simulink model "harmonics"  (Simulink 7.0)
settings: Solver=ode23  StartTime=0.0  StopTime=0.08  RelTol=1e-3
undefined symbols (not defined in the file): D1, Delta
libraries: powerlib x26, powerlib_extras x10
settings Model: Creator=dell  LastModifiedBy=prashik nagdive

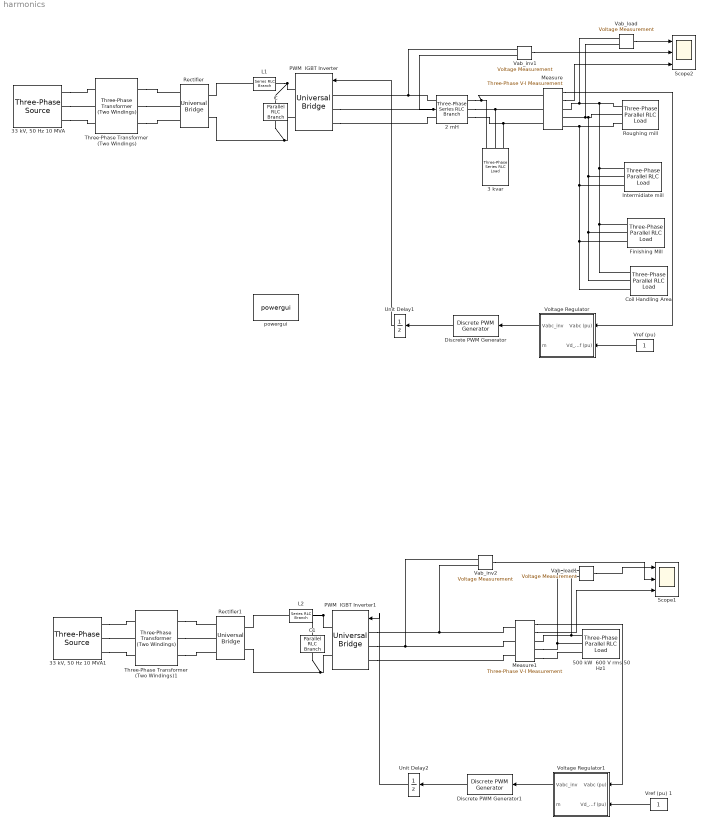
== system harmonics ==
  "2 mH " : powerlib/Elements/Three-Phase Series RLC Branch  DialogController=POWERSYS.PowerSysDialog  PhysicalDomain=powersysdomain  SubClassName=unknown  LeftPortType=p1  RightPortType=p1  LConnTagsString=A|B|C  RConnTagsString=A|B|C  BranchType=L  Resistance=1.0  Inductance=1e-3  Capacitance=1.0  Measurements=None
  3 kvar : powerlib/Elements/Three-Phase Series RLC Load  Orientation=down  DialogController=POWERSYS.PowerSysDialog  PhysicalDomain=powersysdomain  SubClassName=unknown  LeftPortType=p1  RightPortType=p1  LConnTagsString=A|B|C  Configuration=Y (grounded)  NominalVoltage=600  NominalFrequency=50  ActivePower=0  InductivePower=0  CapacitivePower=60e3  Measurements=None
  "33 kV, 50 Hz 10 MVA" : powerlib/Electrical Sources/Three-Phase Source  DialogController=POWERSYS.PowerSysDialog  SystemSampleTime=-1  Voltage=33e3  PhaseAngle=0  Frequency=50  InternalConnection=Yg  SpecifyImpedance=on  Resistance=25e3^2/10e6/5  Inductance=25e3^2/10e6/377  ShortCircuitLevel=10e6  BaseVoltage=33e3  XRratio=5
  "33 kV, 50 Hz 10 MVA1" : powerlib/Electrical Sources/Three-Phase Source  DialogController=POWERSYS.PowerSysDialog  SystemSampleTime=-1  Voltage=33e3  PhaseAngle=0  Frequency=50  InternalConnection=Yg  SpecifyImpedance=on  Resistance=25e3^2/10e6/5  Inductance=25e3^2/10e6/377  ShortCircuitLevel=10e6  BaseVoltage=33e3  XRratio=5
  500 kW  600 V rms 50 Hz1 : powerlib/Elements/Three-Phase Parallel RLC Load  DialogController=POWERSYS.PowerSysDialog  PhysicalDomain=powersysdomain  SubClassName=unknown  LeftPortType=p1  RightPortType=p1  LConnTagsString=A|B|C  Configuration=Y (grounded)  NominalVoltage=600  NominalFrequency=50  ActivePower=500e3  InductivePower=0  CapacitivePower=0  Measurements=Branch voltages and currents
  C : powerlib/Elements/Parallel RLC Branch  Orientation=down  DialogController=POWERSYS.PowerSysDialog  PhysicalDomain=powersysdomain  SubClassName=unknown  LeftPortType=p1  RightPortType=p1  LConnTagsString=a  RConnTagsString=__new0  BranchType=C  Resistance=1.0  Inductance=1.0  SetiL0=off  InitialCurrent=0  Capacitance=5000e-06  Setx0=off  InitialVoltage=0  Measurements=None
  C1 : powerlib/Elements/Parallel RLC Branch  Orientation=down  DialogController=POWERSYS.PowerSysDialog  PhysicalDomain=powersysdomain  SubClassName=unknown  LeftPortType=p1  RightPortType=p1  LConnTagsString=a  RConnTagsString=__new0  BranchType=C  Resistance=1.0  Inductance=1.0  SetiL0=off  InitialCurrent=0  Capacitance=5000e-06  Setx0=off  InitialVoltage=0  Measurements=None
  "Coil Handling Area " : powerlib/Elements/Three-Phase Parallel RLC Load  DialogController=POWERSYS.PowerSysDialog  PhysicalDomain=powersysdomain  SubClassName=unknown  LeftPortType=p1  RightPortType=p1  LConnTagsString=A|B|C  Configuration=Y (grounded)  NominalVoltage=600  NominalFrequency=50  ActivePower=500e3  InductivePower=0  CapacitivePower=0  Measurements=Branch voltages and currents
  Discrete PWM Generator : powerlib_extras/Discrete  Control Blocks/Discrete PWM Generator  Orientation=left  DialogController=POWERSYS.PowerSysDialog  SystemSampleTime=-1  GeneratorMode="3-arm  bridge (6 pulses)"  Fc=2000  Ts=2e-006  Internal=off  mIndex=0.4  Freq=60  Phase=0
  Discrete PWM Generator1 : powerlib_extras/Discrete  Control Blocks/Discrete PWM Generator  Orientation=left  DialogController=POWERSYS.PowerSysDialog  SystemSampleTime=-1  GeneratorMode="3-arm  bridge (6 pulses)"  Fc=2000  Ts=2e-006  Internal=off  mIndex=0.4  Freq=60  Phase=0
  "Finishing Mill " : powerlib/Elements/Three-Phase Parallel RLC Load  DialogController=POWERSYS.PowerSysDialog  PhysicalDomain=powersysdomain  SubClassName=unknown  LeftPortType=p1  RightPortType=p1  LConnTagsString=A|B|C  Configuration=Y (grounded)  NominalVoltage=600  NominalFrequency=50  ActivePower=500e3  InductivePower=0  CapacitivePower=0  Measurements=Branch voltages and currents
  Intermidiate mill : powerlib/Elements/Three-Phase Parallel RLC Load  DialogController=POWERSYS.PowerSysDialog  PhysicalDomain=powersysdomain  SubClassName=unknown  LeftPortType=p1  RightPortType=p1  LConnTagsString=A|B|C  Configuration=Y (grounded)  NominalVoltage=600  NominalFrequency=50  ActivePower=500e3  InductivePower=0  CapacitivePower=0  Measurements=Branch voltages and currents
  L1 : powerlib/Elements/Series RLC Branch  DialogController=POWERSYS.PowerSysDialog  PhysicalDomain=powersysdomain  SubClassName=unknown  LeftPortType=p1  RightPortType=p1  LConnTagsString=__new0  RConnTagsString=__new0  BranchType=L  Resistance=1.0  Inductance=200e-6  SetiL0=off  InitialCurrent=0  Capacitance=1.0  Setx0=off  InitialVoltage=0  Measurements=None
  L2 : powerlib/Elements/Series RLC Branch  DialogController=POWERSYS.PowerSysDialog  PhysicalDomain=powersysdomain  SubClassName=unknown  LeftPortType=p1  RightPortType=p1  LConnTagsString=__new0  RConnTagsString=__new0  BranchType=L  Resistance=1.0  Inductance=200e-6  SetiL0=off  InitialCurrent=0  Capacitance=1.0  Setx0=off  InitialVoltage=0  Measurements=None
  Measure : powerlib/Measurements/Three-Phase V-I Measurement  DialogController=POWERSYS.PowerSysDialog  SystemSampleTime=-1  VoltageMeasurement=phase-to-ground  SetLabelV=off  LabelV=V1  Vpu=on  CurrentMeasurement=yes  SetLabelI=off  LabelI=I1  Ipu=on  Pbase=500e3  Vbase=600  OutputType=Magnitude  PhasorSimulation=off  PSBequivalent=0
  Measure1 : powerlib/Measurements/Three-Phase V-I Measurement  DialogController=POWERSYS.PowerSysDialog  SystemSampleTime=-1  VoltageMeasurement=phase-to-ground  SetLabelV=off  LabelV=V1  Vpu=on  CurrentMeasurement=yes  SetLabelI=off  LabelI=I1  Ipu=on  Pbase=500e3  Vbase=600  OutputType=Magnitude  PhasorSimulation=off  PSBequivalent=0
  PWM  IGBT Inverter : powerlib/Power Electronics/Universal Bridge  Orientation=left  DialogController=POWERSYS.PowerSysDialog  SystemSampleTime=-1  Arms=3  SnubberResistance=5000  SnubberCapacitance=inf  Device=IGBT / Diodes  Ron=1e-3  Lon=0  ForwardVoltages="[  0.0  0.0  ]"  ForwardVoltage=.8  GTOparameters=[ 1e-6 ,1e-6 ]  IGBTparameters=[ 1e-6 , 2e-6 ]  Measurements=Device currents  converterType=Rectifier
  PWM  IGBT Inverter1 : powerlib/Power Electronics/Universal Bridge  Orientation=left  DialogController=POWERSYS.PowerSysDialog  SystemSampleTime=-1  Arms=3  SnubberResistance=5000  SnubberCapacitance=inf  Device=IGBT / Diodes  Ron=1e-3  Lon=0  ForwardVoltages="[  0.0  0.0  ]"  ForwardVoltage=.8  GTOparameters=[ 1e-6 ,1e-6 ]  IGBTparameters=[ 1e-6 , 2e-6 ]  Measurements=Device currents  converterType=Rectifier
  Rectifier : powerlib/Power Electronics/Universal Bridge  DialogController=POWERSYS.PowerSysDialog  SystemSampleTime=-1  Arms=3  SnubberResistance=100  SnubberCapacitance=0.1e-6  Device=Diodes  Ron=1e-3  Lon=0  ForwardVoltages="[  0.8  0.8  ]"  ForwardVoltage=.8  GTOparameters=[ 10e-6 , 20e-6 ]  IGBTparameters=[ 1e-6 , 2e-6 ]  Measurements=Device currents  converterType=Rectifier
  Rectifier1 : powerlib/Power Electronics/Universal Bridge  DialogController=POWERSYS.PowerSysDialog  SystemSampleTime=-1  Arms=3  SnubberResistance=100  SnubberCapacitance=0.1e-6  Device=Diodes  Ron=1e-3  Lon=0  ForwardVoltages="[  0.8  0.8  ]"  ForwardVoltage=.8  GTOparameters=[ 10e-6 , 20e-6 ]  IGBTparameters=[ 1e-6 , 2e-6 ]  Measurements=Device currents  converterType=Rectifier
  Roughing mill : powerlib/Elements/Three-Phase Parallel RLC Load  DialogController=POWERSYS.PowerSysDialog  PhysicalDomain=powersysdomain  SubClassName=unknown  LeftPortType=p1  RightPortType=p1  LConnTagsString=A|B|C  Configuration=Y (grounded)  NominalVoltage=600  NominalFrequency=50  ActivePower=500e3  InductivePower=0  CapacitivePower=0  Measurements=Branch voltages and currents
  Scope1 : Scope  NumInputPorts=3
      settings: TimeRange=0.09999999999999999  YMin=-570~-5~-5  YMax=-465~5~5
  Scope2 : Scope  NumInputPorts=3
      settings: TimeRange=0.09999999999999999  YMin=-500~-800~-0.75  YMax=500~800~0.75
  Three-Phase Transformer (Two Windings) : powerlib/Elements/Three-Phase Transformer (Two Windings)  DialogController=POWERSYS.PowerSysDialog  SystemSampleTime=-1  Winding1Connection=Y  UNITS=pu  NominalPower=[ 5e6 , 50]  Winding1=[ 33e3 , 0.002 , 0.08 ]  Winding2Connection=Delta (D1)  Winding2=[ 600, 0.002 , 0.08 ]  SetSaturation=off  Rm=500  Lm=500  Saturation=[ 0,0 ; 0.0024,1.2 ; 1.0,1.52 ]  Hysteresis=off  DataFile='hysteresis'  SetInitialFlux=off  InitialFluxes=[ 0.8 , -0.8 , 0.7 ]  Measurements=None  MoreParameters=off  BreakLoop=off  DataType=off  TransfoNumber=1
  Three-Phase Transformer (Two Windings)1 : powerlib/Elements/Three-Phase Transformer (Two Windings)  DialogController=POWERSYS.PowerSysDialog  SystemSampleTime=-1  Winding1Connection=Y  UNITS=pu  NominalPower=[ 5e6 , 50]  Winding1=[ 33e3 , 0.002 , 0.08 ]  Winding2Connection=Delta (D1)  Winding2=[ 600, 0.002 , 0.08 ]  SetSaturation=off  Rm=500  Lm=500  Saturation=[ 0,0 ; 0.0024,1.2 ; 1.0,1.52 ]  Hysteresis=off  DataFile='hysteresis'  SetInitialFlux=off  InitialFluxes=[ 0.8 , -0.8 , 0.7 ]  Measurements=None  MoreParameters=off  BreakLoop=off  DataType=off  TransfoNumber=1
  Unit Delay1 : UnitDelay  Orientation=left  SampleTime=2e-006
  Unit Delay2 : UnitDelay  Orientation=left  SampleTime=2e-006
  Vab_inv1 : powerlib/Measurements/Voltage Measurement  Tag=PoWeRsYsTeMmEaSuReMeNt  DialogController=POWERSYS.PowerSysDialog  SystemSampleTime=-1  PhasorSimulation=off  OutputType=Magnitude  PSBequivalent=0
  Vab_inv2 : powerlib/Measurements/Voltage Measurement  Tag=PoWeRsYsTeMmEaSuReMeNt  DialogController=POWERSYS.PowerSysDialog  SystemSampleTime=-1  PhasorSimulation=off  OutputType=Magnitude  PSBequivalent=0
  Vab_load : powerlib/Measurements/Voltage Measurement  Tag=PoWeRsYsTeMmEaSuReMeNt  DialogController=POWERSYS.PowerSysDialog  SystemSampleTime=-1  PhasorSimulation=off  OutputType=Magnitude  PSBequivalent=0
  Vab_load1 : powerlib/Measurements/Voltage Measurement  Tag=PoWeRsYsTeMmEaSuReMeNt  DialogController=POWERSYS.PowerSysDialog  SystemSampleTime=-1  PhasorSimulation=off  OutputType=Magnitude  PSBequivalent=0
  Voltage Regulator : Subsystem  Orientation=left  mask( Voltage Regulator){Kp=0.4, Ki=500, Ts=2e-006}
      mask prompts: Kp "Proportional gain  Kp:"; Ki "Integral gain Ki:"; Ts "Sample time (s) :"
  Voltage Regulator1 : Subsystem  Orientation=left  mask( Voltage Regulator){Kp=0.4, Ki=500, Ts=2e-006}
      mask prompts: Kp "Proportional gain  Kp:"; Ki "Integral gain Ki:"; Ts "Sample time (s) :"
  "Vref (pu) " : Constant  Orientation=left  OutDataType=sfix(16)  OutScaling=2^0
  Vref (pu) 1 : Constant  Orientation=left  OutDataType=sfix(16)  OutScaling=2^0
  powergui : powerlib/powergui  SystemSampleTime=-1  SimulationMode=Discrete  SampleTime=2e-006  echomessages=on  RestoreLinks=yes  x0status=blocks  Frange=[0:2:500]  Ylog=off  Xlog=on  ShowGrid=off  save=off  variable=ZData  structure=ScopeData  ZoomFFT=off  StartTime=0.0  cycles=5  DisplayStyle=1  fundamental=50  FreqAxis=off  MaxFrequency=1000  frequencyindice=0  frequencyindicesteady=1  RmsSteady=2  display=off  Ts=0  frequency=50  methode=off  HookPort=off  Interpol=off  SPID=off  FunctionMessages=off
  wires:
  "Vref (pu) "/1 -> Voltage Regulator/2(Vd_ref (pu))
  Measure/1 -> Voltage Regulator/1(Vabc (pu))
  Voltage Regulator/1(Vabc_inv) -> Discrete PWM Generator/1
  Discrete PWM Generator/1 -> Unit Delay1/1
  Unit Delay1/1 -> PWM  IGBT Inverter/1
  Vab_load/1 -> Scope2/1
  Vab_inv1/1 -> Scope2/2
  Vref (pu) 1/1 -> Voltage Regulator1/2(Vd_ref (pu))
  Measure1/1 -> Voltage Regulator1/1(Vabc (pu))
  Voltage Regulator1/1(Vabc_inv) -> Discrete PWM Generator1/1
  Discrete PWM Generator1/1 -> Unit Delay2/1
  Unit Delay2/1 -> PWM  IGBT Inverter1/1
  Vab_load1/1 -> Scope1/1
  Vab_inv2/1 -> Scope1/2
  Measure1/2 -> Scope1/3
  Measure/2 -> Scope2/3
  connections:
  "33 kV, 50 Hz 10 MVA"/RConn1 -- Three-Phase Transformer (Two Windings)/LConn1
  "33 kV, 50 Hz 10 MVA"/RConn2 -- Three-Phase Transformer (Two Windings)/LConn2
  Three-Phase Transformer (Two Windings)/RConn2 -- Rectifier/LConn2
  Rectifier/RConn1 -- L1/LConn1
  C/RConn1 -- Rectifier/RConn2 -- PWM  IGBT Inverter/RConn2
  C/LConn1 -- L1/RConn1 -- PWM  IGBT Inverter/RConn1
  "33 kV, 50 Hz 10 MVA"/RConn3 -- Three-Phase Transformer (Two Windings)/LConn3
  "2 mH "/LConn1 -- PWM  IGBT Inverter/LConn1 -- Vab_inv1/LConn1
  PWM  IGBT Inverter/LConn3 -- "2 mH "/LConn3
  PWM  IGBT Inverter/LConn2 -- "2 mH "/LConn2 -- Vab_inv1/LConn2
  Measure/LConn1 -- "2 mH "/RConn1 -- 3 kvar/LConn1
  Measure/LConn3 -- "2 mH "/RConn3 -- 3 kvar/LConn3
  Measure/LConn2 -- "2 mH "/RConn2 -- 3 kvar/LConn2
  PWM  IGBT Inverter1/RConn2 -- C1/RConn1 -- Rectifier1/RConn2
  PWM  IGBT Inverter1/RConn1 -- C1/LConn1 -- L2/RConn1
  Vab_load1/LConn2 -- Measure1/RConn1 -- 500 kW  600 V rms 50 Hz1/LConn1
  Vab_load1/LConn1 -- Measure1/RConn2 -- 500 kW  600 V rms 50 Hz1/LConn2
  Measure1/RConn3 -- 500 kW  600 V rms 50 Hz1/LConn3
  Rectifier1/RConn1 -- L2/LConn1
  PWM  IGBT Inverter1/LConn1 -- Measure1/LConn1 -- Vab_inv2/LConn2
  PWM  IGBT Inverter1/LConn2 -- Measure1/LConn2 -- Vab_inv2/LConn1
  PWM  IGBT Inverter1/LConn3 -- Measure1/LConn3
  Roughing mill/LConn2 -- Measure/RConn2 -- Vab_load/LConn2 -- "Coil Handling Area "/LConn2 -- "Finishing Mill "/LConn2 -- Intermidiate mill/LConn2
  Roughing mill/LConn3 -- Measure/RConn3 -- "Coil Handling Area "/LConn3 -- "Finishing Mill "/LConn3 -- Intermidiate mill/LConn3
  Roughing mill/LConn1 -- Measure/RConn1 -- Vab_load/LConn1 -- "Coil Handling Area "/LConn1 -- "Finishing Mill "/LConn1 -- Intermidiate mill/LConn1
  Three-Phase Transformer (Two Windings)/RConn1 -- Rectifier/LConn1
  Three-Phase Transformer (Two Windings)/RConn3 -- Rectifier/LConn3
  "33 kV, 50 Hz 10 MVA1"/RConn1 -- Three-Phase Transformer (Two Windings)1/LConn1
  "33 kV, 50 Hz 10 MVA1"/RConn2 -- Three-Phase Transformer (Two Windings)1/LConn2
  Three-Phase Transformer (Two Windings)1/RConn2 -- Rectifier1/LConn2
  "33 kV, 50 Hz 10 MVA1"/RConn3 -- Three-Phase Transformer (Two Windings)1/LConn3
  Three-Phase Transformer (Two Windings)1/RConn1 -- Rectifier1/LConn1
  Three-Phase Transformer (Two Windings)1/RConn3 -- Rectifier1/LConn3

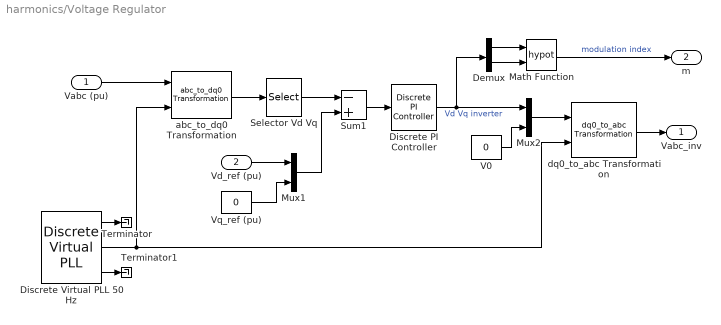
== system harmonics/Voltage Regulator ==
  Vabc (pu) : Inport  OutDataType=sfix(16)  OutScaling=2^0
  Vd_ref (pu) : Inport  Port=2  OutDataType=sfix(16)  OutScaling=2^0
  Demux : Demux  Outputs=2
  Discrete PI Controller : powerlib_extras/Discrete  Control Blocks/Discrete PI Controller  DialogController=POWERSYS.PowerSysDialog  SystemSampleTime=-1  Kp=Kp  Ki=Ki  Par_Limits=[1 -1]  Init=0  Ts=Ts
  Discrete Virtual PLL 50 Hz : powerlib_extras/Discrete  Control Blocks/Discrete Virtual PLL  DialogController=POWERSYS.PowerSysDialog  SystemSampleTime=-1  Freq=50  Phase=0  Ts=Ts
  Math Function : Math  Operator=hypot  OutDataType=sfix(16)  OutScaling=2^0  SaturateOnIntegerOverflow=on
  Mux1 : Mux  Inputs=2
  Mux2 : Mux  Inputs=2
  Selector Vd Vq : Selector  InputPortWidth=3  IndexOptions=Index vector (dialog)  Indices=[1 2]  OutputSizes=1
  Sum1 : Sum  Inputs=-+  OutDataType=sfix(16)  OutScaling=2^0  SaturateOnIntegerOverflow=on  InputSameDT=on
  Terminator : Terminator
  Terminator1 : Terminator
  V0 : Constant  Value=0  OutDataType=sfix(16)  OutScaling=2^0
  Vq_ref (pu) : Constant  Value=0  OutDataType=sfix(16)  OutScaling=2^0
  abc_to_dq0 Transformation : powerlib_extras/Measurements/abc_to_dq0 Transformation  DialogController=POWERSYS.PowerSysDialog  SystemSampleTime=-1
  dq0_to_abc Transformation : powerlib_extras/Measurements/dq0_to_abc Transformation  DialogController=POWERSYS.PowerSysDialog  SystemSampleTime=-1
  Vabc_inv : Outport  OutDataType=sfix(16)  OutScaling=2^0
  m : Outport  Port=2  OutDataType=sfix(16)  OutScaling=2^0
  wires:
  abc_to_dq0 Transformation/1 -> Selector Vd Vq/1
  Vabc (pu)/1 -> abc_to_dq0 Transformation/1
  Selector Vd Vq/1 -> Sum1/1
  Sum1/1 -> Discrete PI Controller/1
  Mux2/1 -> dq0_to_abc Transformation/1
  V0/1 -> Mux2/2
  dq0_to_abc Transformation/1 -> Vabc_inv/1
  Discrete Virtual PLL 50 Hz/2 -> abc_to_dq0 Transformation/2, dq0_to_abc Transformation/2
  Vd_ref (pu)/1 -> Mux1/1
  Vq_ref (pu)/1 -> Mux1/2
  Mux1/1 -> Sum1/2
  Discrete Virtual PLL 50 Hz/1 -> Terminator/1
  Discrete Virtual PLL 50 Hz/3 -> Terminator1/1
  Discrete PI Controller/1 -> Demux/1, Mux2/1  "Vd Vq inverter"
  Demux/1 -> Math Function/1
  Demux/2 -> Math Function/2
  Math Function/1 -> m/1  "modulation index"

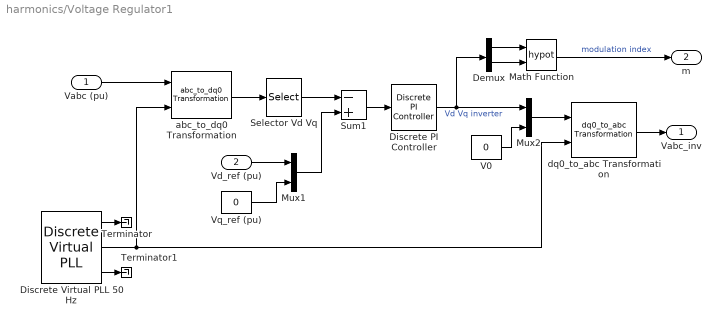
== system harmonics/Voltage Regulator1 ==
  Vabc (pu) : Inport  OutDataType=sfix(16)  OutScaling=2^0
  Vd_ref (pu) : Inport  Port=2  OutDataType=sfix(16)  OutScaling=2^0
  Demux : Demux  Outputs=2
  Discrete PI Controller : powerlib_extras/Discrete  Control Blocks/Discrete PI Controller  DialogController=POWERSYS.PowerSysDialog  SystemSampleTime=-1  Kp=Kp  Ki=Ki  Par_Limits=[1 -1]  Init=0  Ts=Ts
  Discrete Virtual PLL 50 Hz : powerlib_extras/Discrete  Control Blocks/Discrete Virtual PLL  DialogController=POWERSYS.PowerSysDialog  SystemSampleTime=-1  Freq=50  Phase=0  Ts=Ts
  Math Function : Math  Operator=hypot  OutDataType=sfix(16)  OutScaling=2^0  SaturateOnIntegerOverflow=on
  Mux1 : Mux  Inputs=2
  Mux2 : Mux  Inputs=2
  Selector Vd Vq : Selector  InputPortWidth=3  IndexOptions=Index vector (dialog)  Indices=[1 2]  OutputSizes=1
  Sum1 : Sum  Inputs=-+  OutDataType=sfix(16)  OutScaling=2^0  SaturateOnIntegerOverflow=on  InputSameDT=on
  Terminator : Terminator
  Terminator1 : Terminator
  V0 : Constant  Value=0  OutDataType=sfix(16)  OutScaling=2^0
  Vq_ref (pu) : Constant  Value=0  OutDataType=sfix(16)  OutScaling=2^0
  abc_to_dq0 Transformation : powerlib_extras/Measurements/abc_to_dq0 Transformation  DialogController=POWERSYS.PowerSysDialog  SystemSampleTime=-1
  dq0_to_abc Transformation : powerlib_extras/Measurements/dq0_to_abc Transformation  DialogController=POWERSYS.PowerSysDialog  SystemSampleTime=-1
  Vabc_inv : Outport  OutDataType=sfix(16)  OutScaling=2^0
  m : Outport  Port=2  OutDataType=sfix(16)  OutScaling=2^0
  wires:
  abc_to_dq0 Transformation/1 -> Selector Vd Vq/1
  Vabc (pu)/1 -> abc_to_dq0 Transformation/1
  Selector Vd Vq/1 -> Sum1/1
  Sum1/1 -> Discrete PI Controller/1
  Mux2/1 -> dq0_to_abc Transformation/1
  V0/1 -> Mux2/2
  dq0_to_abc Transformation/1 -> Vabc_inv/1
  Discrete Virtual PLL 50 Hz/2 -> abc_to_dq0 Transformation/2, dq0_to_abc Transformation/2
  Vd_ref (pu)/1 -> Mux1/1
  Vq_ref (pu)/1 -> Mux1/2
  Mux1/1 -> Sum1/2
  Discrete Virtual PLL 50 Hz/1 -> Terminator/1
  Discrete Virtual PLL 50 Hz/3 -> Terminator1/1
  Discrete PI Controller/1 -> Demux/1, Mux2/1  "Vd Vq inverter"
  Demux/1 -> Math Function/1
  Demux/2 -> Math Function/2
  Math Function/1 -> m/1  "modulation index"
